simulink model "sampleModel1867_5_sub_sub"  (R2023a)
settings: Solver=VariableStepAuto  StartTime=0.0  StopTime=10.0  RelTol=1e-3
libraries: hdlsllib x7, simulink x3
settings Model: Creator=user1  LastModifiedBy=user1
settings OptimizationCC: BlockReduction=off  ConditionallyExecuteInputs=off

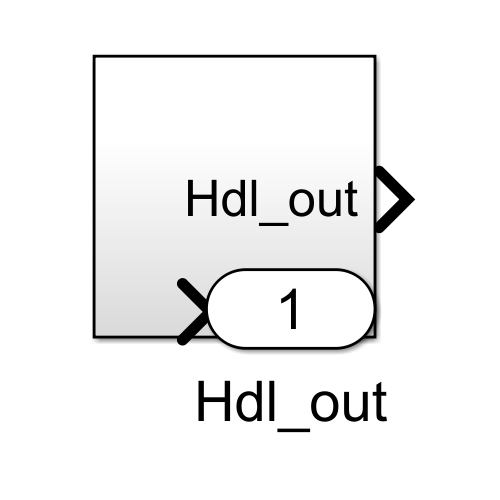
[thumbnail: Simulink's stored preview of the top-level diagram]
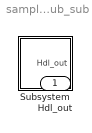
== system sampleModel1867_5_sub_sub ==
  Subsystem : Subsystem
  Hdl_out : Outport  OutDataTypeStr=uint8

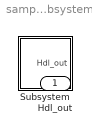
== system sampleModel1867_5_sub_sub/Subsystem ==
  Subsystem : Subsystem
  Hdl_out : Outport  OutDataTypeStr=uint8

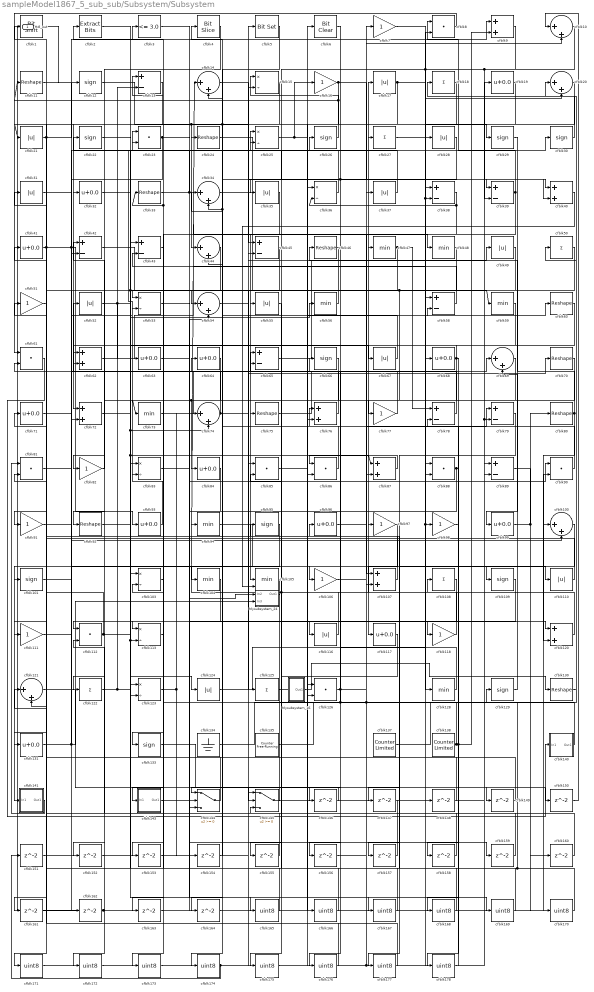
== system sampleModel1867_5_sub_sub/Subsystem/Subsystem ==
  Mysubsystem_16 : Subsystem  TreatAsAtomicUnit=on  RTWFcnName=Mysubsystem_16
      settings: RTWFcnNameOpts=User specified  RTWFileNameOpts=Use function name
  Mysubsystem_24 : Subsystem  TreatAsAtomicUnit=on  RTWFcnName=Mysubsystem_24
      settings: RTWFcnNameOpts=User specified  RTWFileNameOpts=Use function name
  cfblk1 : hdlsllib/Logic and Bit Operations/Bit Shift  mode=Shift Left Logical  N=0
  cfblk{10,14,20,34,44,54,69,74,100,121} (10 alike) : Sum  Inputs=|++  OutDataTypeStr=uint8
  cfblk{12,22,26,29..30,66,95,101,109,129,133} (11 alike) : Signum
  cfblk{15,25,36,53,83,103,113,123} (8 alike) : Product  Inputs=*/  OutDataTypeStr=uint8  RndMeth=Zero  SaturateOnIntegerOverflow=on
  cfblk{47..48,56,59,73,94,104..105,128} (9 alike) : MinMax  OutDataTypeStr=uint8
  cfblk{7,16,51,77,82,91,97..98,106,111,118} (11 alike) : Gain  OutDataTypeStr=uint8
  cfblk{9,40,62,72,76,87,107,120} (8 alike) : Sum  OutDataTypeStr=uint8
  cfblk{18,27,50,108,122,125} (6 alike) : Sum  Inputs=+  OutDataTypeStr=uint8
  cfblk{11,24,33,46,60,70,75,80,92,130} (10 alike) : Reshape
  cfblk{17,21,28,31,35,37,49,52,55,67,110,116,124} (13 alike) : Abs  OutDataTypeStr=uint8  SaturateOnIntegerOverflow=off
  cfblk{8,23,61,81,85..86,88,90,112,126} (10 alike) : DotProduct  OutDataTypeStr=uint8
  cfblk{19,32,41,63..64,68,71,84,93,96,99,117,131} (13 alike) : Bias  Bias=0.0  SaturateOnIntegerOverflow=off
  cfblk{13,38..39,42..43,45,58,65,78..79,89} (11 alike) : Sum  Inputs=+-  OutDataTypeStr=uint8
  cfblk134 : Ground
  cfblk135 : hdlsllib/Sources/Counter Free-Running  NumBits=16  tsamp=-1
  cfblk137 : hdlsllib/Sources/Counter Limited  uplimit=7  tsamp=-1
  cfblk138 : hdlsllib/Sources/Counter Limited  uplimit=7  tsamp=-1
  cfblk140 : Subsystem
      settings: LibrarySourceBlock=|
      | hdlsllib/Ports &
      | Subsystems/Subsystem
  cfblk141 : Subsystem
      settings: LibrarySourceBlock=|
      | hdlsllib/Ports &
      | Subsystems/Subsystem
  cfblk143 : Subsystem
      settings: LibrarySourceBlock=|
      | hdlsllib/Ports &
      | Subsystems/Subsystem
  cfblk144 : Switch  OutDataTypeStr=uint8  SaturateOnIntegerOverflow=off  InputSameDT=off
  cfblk145 : Switch  OutDataTypeStr=uint8  SaturateOnIntegerOverflow=off  InputSameDT=off
  cfblk{146..164} (19 alike) : Delay  SampleTime=1
  cfblk{165..178} (14 alike) : DataTypeConversion  OutDataTypeStr=uint8  SaturateOnIntegerOverflow=off  RndMeth=Floor
  cfblk2 : simulink/Logic and Bit Operations/Extract Bits  bitsToExtract=Upper half  numBits=8  bitIdxRange=[0 7]  outScalingMode=Preserve fixed-point scaling
      settings: LibrarySourceBlock=|
      | hdlsllib/Logic and Bit
      | Operations/Extract Bits
  cfblk3 : hdlsllib/Logic and Bit Operations/Compare To Constant  relop=<=  const=3.0  OutDataTypeStr=uint8
  cfblk4 : hdlsllib/Logic and Bit Operations/Bit Slice  lidx=7  ridx=0
  cfblk5 : simulink/Logic and Bit Operations/Bit Set  iBit=0
      settings: LibrarySourceBlock=|
      | hdlsllib/Logic and Bit
      | Operations/Bit Set
  cfblk6 : simulink/Logic and Bit Operations/Bit Clear  iBit=0
      settings: LibrarySourceBlock=|
      | hdlsllib/Logic and Bit
      | Operations/Bit Clear
  Hdl_out : Outport  OutDataTypeStr=uint8
  wires:
  Mysubsystem_24/1(Out1) -> cfblk148/1
  cfblk63/1 -> Mysubsystem_24/2(In2)
  cfblk40/1 -> Mysubsystem_24/1(In1)
  Mysubsystem_16/1(Out1) -> cfblk130/1
  cfblk178/1 -> cfblk108/1
  cfblk98/1 -> cfblk178/1
  cfblk177/1 -> cfblk126/1
  cfblk108/1 -> cfblk177/1
  cfblk176/1 -> cfblk121/2
  cfblk6/1 -> cfblk176/1
  cfblk175/1 -> cfblk6/1
  cfblk55/1 -> cfblk175/1
  cfblk174/1 -> cfblk38/1, cfblk98/1, cfblk7/1, cfblk151/1
  cfblk173/1 -> cfblk5/1
  cfblk109/1 -> cfblk173/1
  cfblk172/1 -> cfblk89/2
  cfblk104/1 -> cfblk172/1
  cfblk171/1 -> cfblk89/1
  cfblk51/1 -> cfblk171/1
  cfblk170/1 -> cfblk129/1, cfblk97/1
  cfblk169/1 -> cfblk85/2
  cfblk168/1 -> cfblk85/1
  cfblk167/1 -> cfblk43/1
  cfblk85/1 -> cfblk167/1
  cfblk166/1 -> cfblk3/1
  cfblk133/1 -> cfblk166/1
  cfblk165/1 -> cfblk71/1
  cfblk3/1 -> cfblk165/1
  cfblk164/1 -> cfblk45/2
  cfblk163/1 -> cfblk90/2
  cfblk162/1 -> cfblk144/3, Hdl_out/1
  cfblk11/1 -> cfblk162/1
  cfblk161/1 -> cfblk88/1
  cfblk160/1 -> cfblk78/2
  cfblk159/1 -> cfblk1/1
  cfblk53/1 -> cfblk159/1
  cfblk158/1 -> cfblk112/2
  cfblk157/1 -> cfblk44/2
  cfblk100/1 -> cfblk157/1
  cfblk156/1 -> cfblk107/2
  cfblk155/1 -> cfblk123/1
  cfblk117/1 -> cfblk155/1
  cfblk154/1 -> cfblk34/1
  cfblk153/1 -> cfblk54/2
  cfblk113/1 -> cfblk153/1
  cfblk152/1 -> cfblk15/2
  cfblk66/1 -> cfblk152/1
  cfblk151/1 -> cfblk145/1
  cfblk150/1 -> cfblk10/1
  cfblk149/1 -> cfblk103/2
  cfblk83/1 -> cfblk149/1
  cfblk148/1 -> cfblk121/1
  cfblk147/1 -> cfblk145/3
  cfblk79/1 -> cfblk147/1
  cfblk146/1 -> cfblk144/1
  cfblk14/1 -> cfblk40/2
  cfblk12/1 -> cfblk45/1
  cfblk7/1 -> cfblk20/2
  cfblk38/1 -> cfblk36/2, cfblk87/2
  cfblk123/1 -> cfblk74/1, cfblk154/1
  cfblk86/1 -> cfblk25/1
  cfblk69/1 -> cfblk126/2
  cfblk145/1 -> cfblk79/2, cfblk19/1
  cfblk78/1 -> cfblk61/2
  cfblk143/1(Out1) -> cfblk90/1
  cfblk96/1 -> cfblk10/2
  cfblk130/1 -> cfblk20/1
  cfblk58/1 -> cfblk43/2
  cfblk9/1 -> cfblk35/1
  cfblk73/1 -> cfblk36/1
  cfblk32/1 -> cfblk113/2, cfblk169/1
  cfblk103/1 -> cfblk83/2
  cfblk59/1 -> cfblk112/1
  cfblk128/1 -> cfblk96/1
  cfblk129/1 -> cfblk69/2
  cfblk18/1 -> cfblk86/2
  cfblk54/1 -> cfblk47/1
  cfblk71/1 -> cfblk69/1
  cfblk140/1(Out1) -> cfblk76/1, cfblk95/1
  cfblk23/1 -> cfblk72/2, cfblk120/1
  cfblk67/1 -> cfblk23/1, cfblk34/2
  cfblk27/1 -> cfblk29/1
  cfblk107/1 -> cfblk41/1
  cfblk31/1 -> cfblk109/1
  cfblk89/1 -> cfblk170/1
  cfblk106/1 -> cfblk79/1
  cfblk88/1 -> cfblk118/1, cfblk164/1
  cfblk45/1 -> cfblk143/1(In1)
  cfblk81/1 -> cfblk100/2
  cfblk52/1 -> cfblk67/1, cfblk63/1
  cfblk75/1 -> cfblk8/2
  cfblk77/1 -> cfblk51/1
  cfblk2/1 -> cfblk87/1, cfblk150/1, cfblk59/1
  cfblk126/1 -> cfblk66/1, cfblk58/2
  cfblk74/1 -> cfblk70/1, cfblk62/2
  cfblk122/1 -> cfblk27/1, cfblk13/2
  cfblk80/1 -> cfblk46/1, cfblk120/2
  cfblk135/1 -> cfblk37/1, cfblk58/1
  cfblk43/1 -> cfblk113/1
  cfblk94/1 -> cfblk106/1
  cfblk33/1 -> cfblk128/1, cfblk25/2
  cfblk29/1 -> cfblk99/1
  cfblk64/1 -> cfblk84/1, cfblk73/1
  cfblk47/1 -> cfblk131/1, cfblk78/1
  cfblk22/1 -> cfblk83/1
  cfblk50/1 -> cfblk77/1, cfblk76/2
  cfblk19/1 -> cfblk54/1, cfblk111/1
  cfblk34/1 -> cfblk107/1
  cfblk116/1 -> cfblk4/1
  cfblk112/1 -> cfblk31/1, cfblk124/1
  cfblk62/1 -> cfblk28/1
  cfblk15/1 -> cfblk24/1, cfblk21/1
  cfblk91/1 -> cfblk26/1
  cfblk84/1 -> cfblk144/2
  cfblk68/1 -> cfblk62/1, cfblk122/1, cfblk158/1
  cfblk24/1 -> cfblk48/1
  cfblk26/1 -> cfblk15/1, cfblk11/1
  cfblk134/1 -> cfblk100/1
  cfblk101/1 -> cfblk53/2
  cfblk28/1 -> cfblk104/1, cfblk156/1
  cfblk1/1 -> cfblk12/1
  cfblk10/1 -> cfblk88/2, cfblk38/2, cfblk146/1, cfblk39/2
  cfblk17/1 -> cfblk44/1, cfblk39/1
  cfblk16/1 -> cfblk40/1, cfblk123/2
  cfblk39/1 -> cfblk8/1, cfblk163/1
  cfblk125/1 -> cfblk60/1
  cfblk111/1 -> cfblk42/2
  cfblk110/1 -> cfblk81/2
  cfblk61/1 -> cfblk140/1(In1)
  cfblk97/1 -> cfblk117/1
  cfblk4/1 -> cfblk92/1
  cfblk105/1 -> cfblk133/1
  cfblk138/1 -> cfblk9/2, cfblk168/1, cfblk13/1
  cfblk21/1 -> cfblk101/1, cfblk9/1
  cfblk20/1 -> cfblk32/1
  cfblk42/1 -> cfblk125/1
  cfblk30/1 -> cfblk18/1
  cfblk92/1 -> cfblk56/1, cfblk74/2
  cfblk124/1 -> cfblk68/1
  cfblk49/1 -> cfblk94/1
  cfblk121/1 -> cfblk145/2
  cfblk137/1 -> cfblk50/1
  cfblk82/1 -> cfblk42/1
  cfblk141/1(Out1) -> cfblk81/1
  cfblk36/1 -> cfblk22/1
  cfblk37/1 -> cfblk14/2
  cfblk56/1 -> cfblk55/1
  cfblk76/1 -> cfblk52/1
  cfblk90/1 -> cfblk64/1
  cfblk35/1 -> cfblk75/1
  cfblk95/1 -> cfblk141/1(In1)
  cfblk44/1 -> cfblk91/1
  cfblk70/1 -> cfblk82/1
  cfblk48/1 -> cfblk116/1
  cfblk144/1 -> cfblk33/1, cfblk23/2
  cfblk131/1 -> Mysubsystem_24/3(In3), cfblk65/1
  cfblk93/1 -> cfblk2/1
  cfblk46/1 -> cfblk53/1
  cfblk118/1 -> cfblk17/1
  cfblk72/1 -> cfblk103/1
  cfblk120/1 -> cfblk14/1, cfblk65/2
  cfblk65/1 -> cfblk49/1
  cfblk60/1 -> cfblk105/1
  cfblk13/1 -> cfblk72/1
  cfblk8/1 -> cfblk61/1
  cfblk41/1 -> cfblk93/1, cfblk30/1, cfblk161/1
  cfblk5/1 -> cfblk174/1
  cfblk25/1 -> cfblk16/1, cfblk110/1
  cfblk99/1 -> cfblk80/1, cfblk160/1
  cfblk87/1 -> cfblk86/1

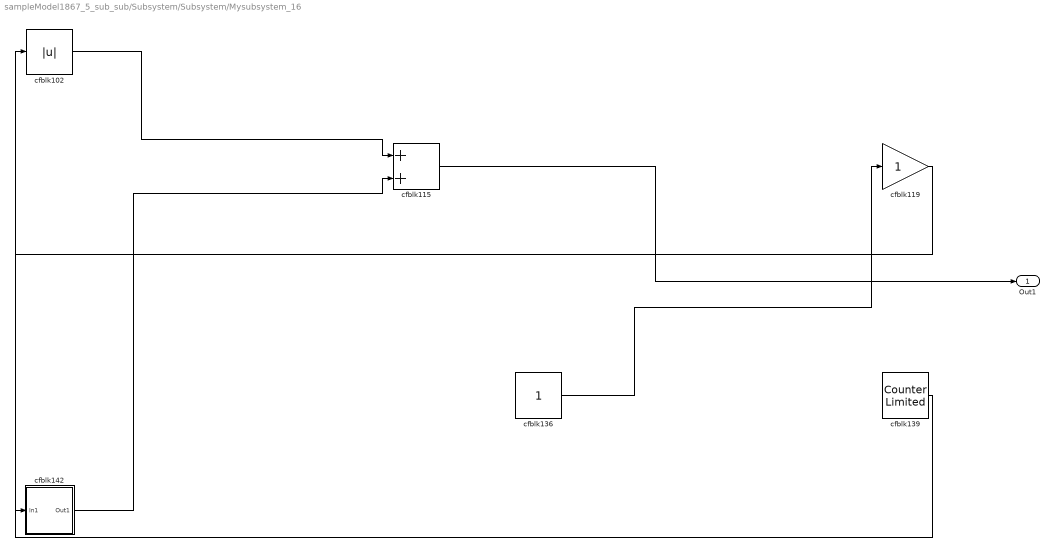
== system sampleModel1867_5_sub_sub/Subsystem/Subsystem/Mysubsystem_16 ==
  cfblk102 : Abs  SaturateOnIntegerOverflow=off
  cfblk115 : Sum
  cfblk119 : Gain
  cfblk136 : Constant  SampleTime=-1
  cfblk139 : hdlsllib/Sources/Counter Limited  uplimit=7  tsamp=-1
  cfblk142 : Subsystem
      settings: LibrarySourceBlock=|
      | hdlsllib/Ports &
      | Subsystems/Subsystem
  Out1 : Outport
  wires:
  cfblk119/1 -> cfblk142/1(In1)
  cfblk142/1(Out1) -> cfblk115/2
  cfblk136/1 -> cfblk119/1
  cfblk115/1 -> Out1/1
  cfblk139/1 -> cfblk102/1
  cfblk102/1 -> cfblk115/1

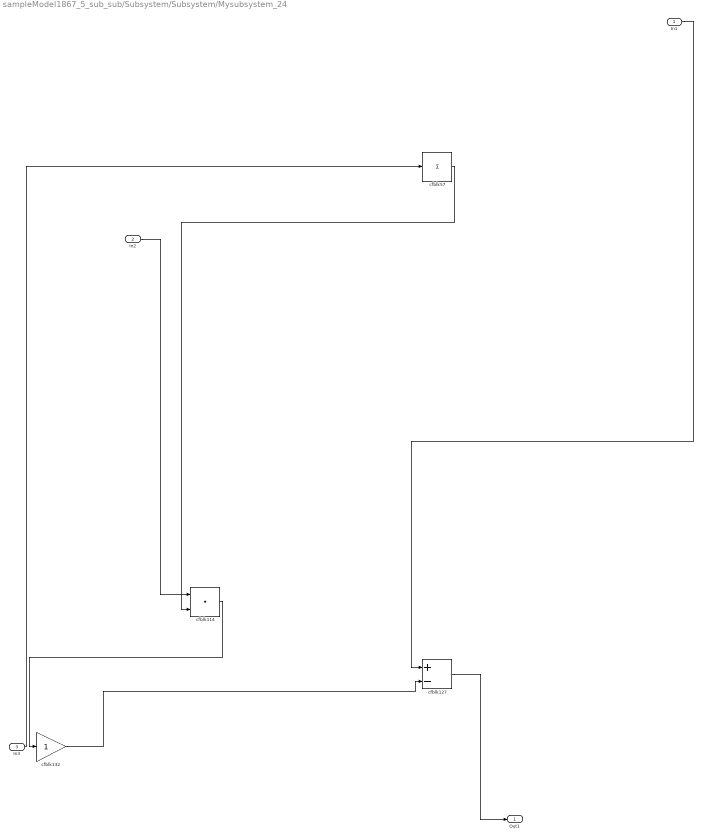
== system sampleModel1867_5_sub_sub/Subsystem/Subsystem/Mysubsystem_24 ==
  In1 : Inport
  In2 : Inport  Port=2
  In3 : Inport  Port=3
  cfblk114 : DotProduct  OutDataTypeStr=Inherit: Inherit via internal rule
  cfblk127 : Sum  Inputs=+-
  cfblk132 : Gain
  cfblk57 : Sum  Inputs=+
  Out1 : Outport
  wires:
  In3/1 -> cfblk57/1
  cfblk57/1 -> cfblk114/2
  cfblk114/1 -> cfblk132/1
  cfblk127/1 -> Out1/1
  cfblk132/1 -> cfblk127/2
  In2/1 -> cfblk114/1
  In1/1 -> cfblk127/1

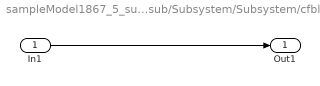
== system sampleModel1867_5_sub_sub/Subsystem/Subsystem/cfblk140 ==
  In1 : Inport
  Out1 : Outport
  wires:
  In1/1 -> Out1/1

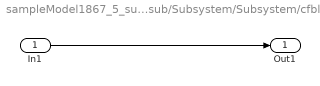
== system sampleModel1867_5_sub_sub/Subsystem/Subsystem/cfblk141 ==
  In1 : Inport
  Out1 : Outport
  wires:
  In1/1 -> Out1/1

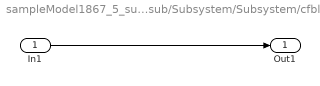
== system sampleModel1867_5_sub_sub/Subsystem/Subsystem/cfblk143 ==
  In1 : Inport
  Out1 : Outport
  wires:
  In1/1 -> Out1/1

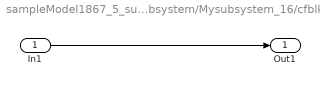
== system sampleModel1867_5_sub_sub/Subsystem/Subsystem/Mysubsystem_16/cfblk142 ==
  In1 : Inport
  Out1 : Outport
  wires:
  In1/1 -> Out1/1
